simulink model "sldrt_newtest_2025b"  (R2025b)
settings: Solver=FixedStepDiscrete  StartTime=0.0  StopTime=inf  FixedStep=0.02  RelTol=1e-3  EnableMultiTasking=on
PreLoadFcn:
  | setup_buses
  | FromApp_Template = Simulink.Bus.createMATLABStruct('FromAppBus_Type');
  | assignin('base', 'FromApp_Template', FromApp_Template);
model workspace (MAT data in the model file):
  AppAirBtn = Simulink.Parameter
  AppAirBtn.Value = 0
  AppAirBtn.Complexity = 'real'
  AppAirBtn.Dimensions = [1 1]
  AppAirBtn.DataType = 'boolean'
  AppAmplitude = Simulink.Parameter
  AppAmplitude.Value = 800
  AppAmplitude.Complexity = 'real'
  AppAmplitude.Dimensions = [1 1]
  AppAmplitude.DataType = 'auto'
  AppPeriods = Simulink.Parameter
  AppPeriods.Value = 2
  AppPeriods.Complexity = 'real'
  AppPeriods.Dimensions = [1 1]
  AppPeriods.DataType = 'auto'
  AppSharpness = Simulink.Parameter
  AppSharpness.Value = 2
  AppSharpness.Complexity = 'real'
  AppSharpness.Dimensions = [1 1]
  AppSharpness.DataType = 'auto'
  AppZeroBtn = Simulink.Parameter
  AppZeroBtn.Value = 0
  AppZeroBtn.Complexity = 'real'
  AppZeroBtn.Dimensions = [1 1]
  AppZeroBtn.DataType = 'boolean'
  Code = Simulink.Parameter
  Code.Value = 279.564441178
  Code.Complexity = 'real'
  Code.Dimensions = [1 1]
  Code.DataType = 'auto'
  CodeScaleCoeff = Simulink.Parameter
  CodeScaleCoeff.Value = 0.0214546484044
  CodeScaleCoeff.Complexity = 'real'
  CodeScaleCoeff.Dimensions = [1 1]
  CodeScaleCoeff.DataType = 'auto'
  SignalToDAC = Simulink.Parameter
  SignalToDAC.Value = [2048 2048 2049 2049 2050 2050 2050 2051 2051 2051 2052 2052 ... (20000 elements, 1x20000)]
  SignalToDAC.Complexity = 'real'
  SignalToDAC.Dimensions = [1 20000]
  SignalToDAC.DataType = 'uint16'
  myLUTobj = Simulink.LookupTable
  myLUTobj.Table = Simulink.lookuptable.Table
  myLUTobj.Table.Value = [1 2 3 4 5 6 7 8 9 10]
  myLUTobj.Table.Dimensions = [1 10]
  myLUTobj.Table.DataType = 'auto'
  myLUTobj.Table.FieldName = 'V'
  myLUTobj.Breakpoints = Simulink.lookuptable.Breakpoint
  myLUTobj.Breakpoints.Value = [1 2 3 4 5 6 7 8 9 10]
  myLUTobj.Breakpoints.TunableSizeName = 'N1'
  myLUTobj.Breakpoints.TunableSizeValue = -1
  myLUTobj.Breakpoints.Dimensions = [1 10]
  myLUTobj.Breakpoints.DataType = 'auto'
  myLUTobj.Breakpoints.FieldName = 'Value'
  myLUTobj.AllowMultipleInstancesOfTypeToHaveDifferentTableBreakpointSizes = 0
  myLUTobj.SupportTunableSize = 1
  myLUTobj.StructTypeInfo = Simulink.lookuptable.StructTypeInfo
  myLUTobj.StructTypeInfo.Name = 'myLUTstruct'
  myLUTobj.StructTypeInfo.DataScope = 'Auto'
  xx = Simulink.Parameter
  xx.Value = [41343 41343.1 41343.2 41343.3 41343.4 41343.5 41343.6 41343.7 41343.8 41343.9 41344 41682 41973 42429 43533 44717 46388 47769 49334 50678 51343 53185 55663 57862 60000]
  xx.Complexity = 'real'
  xx.Dimensions = [1 25]
  xx.DataType = 'auto'
  yy = Simulink.Parameter
  yy.Value = [3122 3121.9 3121.8 3121.7 3121.6 3121.5 3121.4 3121.3 3121.2 3121.1 3121 2440 1964 1465 976 698 466 335 232 181 154 103 51 20 0]
  yy.Complexity = 'real'
  yy.Dimensions = [1 25]
  yy.DataType = 'auto'
libraries: simulink x7, simulink_extras x4, dspnetwork x2, dspstat3 x2, etargetslib x1
settings Model: ExplicitPartitioning=on  Creator=Huawei  LastModifiedBy=lolve
settings SolverCC: AlgebraicLoopSolver=TrustRegion  AutoInsertRateTranBlk=on  DecoupledContinuousIntegration=on  MinimalZcImpactIntegration=on
settings DataIOCC: ExternalInput=TestInput
settings OptimizationCC: BlockReduction=off  DefaultParameterBehavior=Inlined  UseDivisionForNetSlopeComputation=on  GainParamInheritBuiltInType=on  UseFloatMulNetSlope=on  InlineInvariantSignals=on  OptimizeBlockIOStorage=off  BufferReuse=off  ReuseModelBlockBuffer=off  GlobalBufferReuse=off  ExpressionFolding=off  EnableMemcpy=off  PassReuseOutputArgsThreshold=0.0  LocalBlockOutputs=off  EfficientFloat2IntCast=on  MaxStackSize=64  OptimizeDataStoreBuffers=off  BusAssignmentInplaceUpdate=off  OptimizationLevel=level0  OptimizationCustomize=off
settings DebuggingCC: ParameterTunabilityLossMsg=error  UnconnectedInputMsg=warning  UnconnectedOutputMsg=warning  UnconnectedLineMsg=warning  ArithmeticOperatorsInVariantConditions=warning
settings HardwareCC: ProdBitPerLong=64.0  ProdHWDeviceType=Intel->x86-64 (Linux 64)
settings ModelReferenceCC: EnableRefExpFcnMdlSchedulingChecks=on
settings SFSimCC: SimUseLocalCustomCode=off  MATLABDynamicMemAlloc=off  CustomCodeUndefinedFunction=UseInterfaceOnly
settings RTWCC: SystemTargetFile=sldrt.tlc  TemplateMakefile=sldrt.tmf  GenerateReport=on  RTWUseLocalCustomCode=off  Toolchain=Microsoft Visual C++ 2022 v17.0 | nmake (64-bit Windows)  LaunchReport=on  RTWCompilerOptimization=on  GPUComputeCapability=3.5  DLArmComputeVersion=19.05  Description=Simulink Desktop Real-Time
settings CodeAppCC: ForceParamTrailComments=on  MaxIdLength=95.0  OperatorAnnotations=on
settings SimulinkDesktopRealTimeCC: ExtModeTransport=0.0  ExtModeStaticAllocSize=1000000.0  TargetLibSuffix=_sldrt.a  TargetPreCompLibLocation=D:\MATLAB\R2025b\toolbox\sldrt\lib\win64  MultiwordLength=2048.0  DynamicStringBufferSize=256.0  ParMdlRefBuildCompliant=on  PreserveMATLABNamespacesInGeneratedCode=on  SubcomponentCodeInterfacePackaging=Reusable function

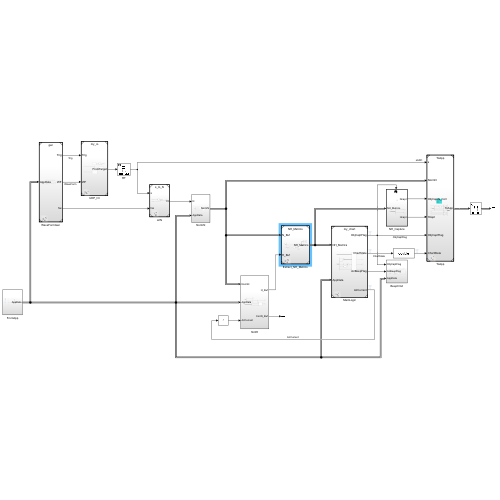
[thumbnail: Simulink's stored preview of the top-level diagram]
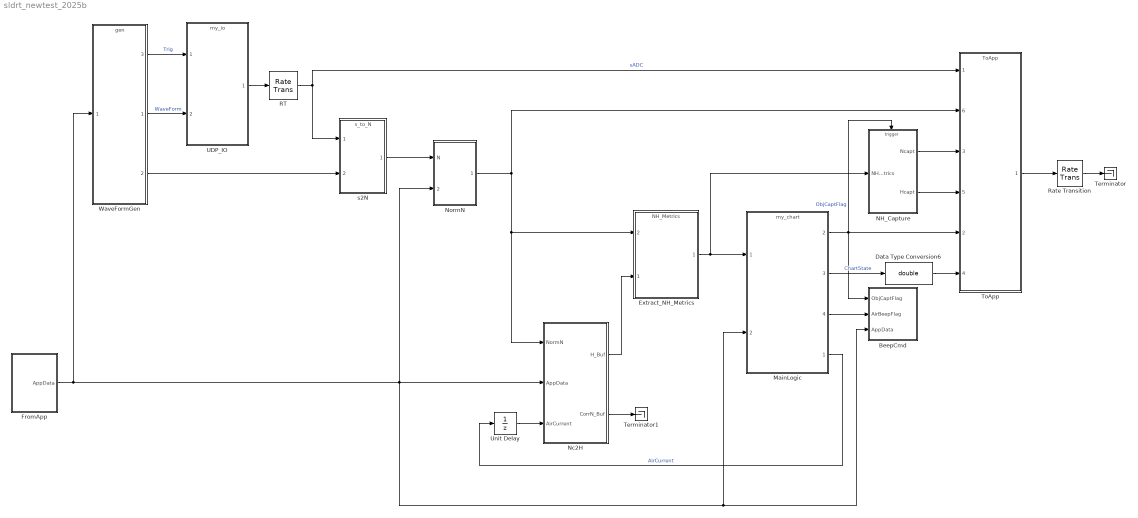
== system sldrt_newtest_2025b ==
  BeepCmd : Subsystem
  Data Type Conversion6 : DataTypeConversion  OutDataTypeStr=double  SaturateOnIntegerOverflow=off  RndMeth=Floor
  Extract_NH_Metrics : ModelReference  ModelNameDialog=NH_Metrics  SimulationMode=Normal  ModelReferenceVersion=1.50
      settings: PortSchema="{\"entries\":[{\"content\":{\"sides\":[{\"content\":{\"connectorIds\":[\"In2\",\"In1\"]},\"type\":\"ConnectorPlacement.EquallySpacedRectSide\",\"uuid\":\"3a38ccda-2223-4b10-94c8-e18dfc340c6f\"},{\"content\":{\"connectorIds\":[\"Out1\"],\"side\":\"RIGHT\"},\"type\":\"ConnectorPlacement.EquallySpacedRectSide\",\"uuid\":\"8419e0ff-c5db-4e1e-bcd8-780560147c58\"},{\"content\":{\"side\":\"TOP\"},\"type\":\"ConnectorPlacement.EquallySpacedRectSide\",\"uuid\":\"08e19ae9-9d85-4fd9-806d-4003401e858c\"}]},\"type\":\"ConnectorPlacement.EquallySpacedConnector\",\"uuid\":\"799394af-d852-43f2-8721-bc316fb3f3ae\"}],\"packageUris\":[\"http://schema.mathworks.com/mf0/Connector/R2020b\"],\"version\":\"1.0\"}"
  FromApp : Subsystem
  MainLogic : ModelReference  Priority=2  ModelNameDialog=my_chart.slx  SimulationMode=Normal  ScheduleRatesWith=Schedule Editor  ModelReferenceVersion=1.246
      settings: PortSchema="{\"entries\":[{\"content\":{\"sides\":[{\"content\":{\"connectorIds\":[\"In1\",\"In2\"]},\"type\":\"ConnectorPlacement.EquallySpacedRectSide\",\"uuid\":\"0ee1a6e0-4898-4e5e-a3f2-a4873c516c9b\"},{\"content\":{\"connectorIds\":[\"Out2\",\"Out3\",\"Out4\",\"Out1\"],\"side\":\"RIGHT\"},\"type\":\"ConnectorPlacement.EquallySpacedRectSide\",\"uuid\":\"631dc309-49f9-48aa-93e0-96384f954726\"},{\"content\":{\"side\":\"TOP\"},\"type\":\"ConnectorPlacement.EquallySpacedRectSide\",\"uuid\":\"941348e0-d81f-4f79-b9d4-bd78ea26c6c3\"}]},\"type\":\"ConnectorPlacement.EquallySpacedConnector\",\"uuid\":\"94e2f426-079c-4c5f-a540-67617520c55b\"}],\"packageUris\":[\"http://schema.mathworks.com/mf0/Connector/R2020b\"],\"version\":\"1.0\"}"
  NH_Capture : Subsystem
  Nc2H : Subsystem
  NormN : Subsystem
  RT : RateTransition  Integrity=off  Deterministic=off  OutPortSampleTime=0.02
  Rate Transition : RateTransition
  Terminator : Terminator
  Terminator1 : Terminator
  ToApp : ModelReference  ModelNameDialog=ToApp.slx  SimulationMode=Normal  ModelReferenceVersion=1.41
      settings: PortSchema="{\"entries\":[{\"content\":{\"sides\":[{\"content\":{\"connectorIds\":[\"In1\",\"In6\",\"In3\",\"In5\",\"In2\",\"In4\"]},\"type\":\"ConnectorPlacement.EquallySpacedRectSide\",\"uuid\":\"2a60f3ad-f22a-481e-bfa0-3f1feb70fa0e\"},{\"content\":{\"connectorIds\":[\"Out1\"],\"side\":\"RIGHT\"},\"type\":\"ConnectorPlacement.EquallySpacedRectSide\",\"uuid\":\"a97ccfa7-4022-4d86-888c-0861d8007155\"},{\"content\":{\"side\":\"TOP\"},\"type\":\"ConnectorPlacement.EquallySpacedRectSide\",\"uuid\":\"d2721f0e-98b2-48c2-b67a-f5bd578bfe97\"}]},\"type\":\"ConnectorPlacement.EquallySpacedConnector\",\"uuid\":\"dadb772c-2c9f-4732-9bcd-da2802ebc2cf\"}],\"packageUris\":[\"http://schema.mathworks.com/mf0/Connector/R2020b\"],\"version\":\"1.0\"}"
  UDP_IO : ModelReference  ModelNameDialog=my_io.slx  SimulationMode=Normal  ModelReferenceVersion=1.32
  Unit Delay : UnitDelay  InitialCondition=1  SampleTime=-1  HasFrameUpgradeWarning=on
  WaveFormGen : ModelReference  ModelNameDialog=gen.slx  SimulationMode=Normal  ModelReferenceVersion=1.31
      settings: PortSchema="{\"entries\":[{\"content\":{\"sides\":[{\"content\":{\"connectorIds\":[\"In1\"]},\"type\":\"ConnectorPlacement.EquallySpacedRectSide\",\"uuid\":\"6ec36bc1-2d75-43bf-b54c-2c7b61273d73\"},{\"content\":{\"connectorIds\":[\"Out3\",\"Out1\",\"Out2\"],\"side\":\"RIGHT\"},\"type\":\"ConnectorPlacement.EquallySpacedRectSide\",\"uuid\":\"17382908-6507-41c0-8990-8a468161a0d7\"},{\"content\":{\"side\":\"TOP\"},\"type\":\"ConnectorPlacement.EquallySpacedRectSide\",\"uuid\":\"0c9326df-e88c-4f4a-83e1-d6c039129936\"}]},\"type\":\"ConnectorPlacement.EquallySpacedConnector\",\"uuid\":\"e56dde6f-bf8e-407c-8fff-cfa8939317ce\"}],\"packageUris\":[\"http://schema.mathworks.com/mf0/Connector/R2020b\"],\"version\":\"1.0\"}"
  s2N : ModelReference  ModelNameDialog=s_to_N.slx  SimulationMode=Normal  ModelReferenceVersion=1.5
  wires:
  UDP_IO/1 -> RT/1
  WaveFormGen/1 -> UDP_IO/2  "WaveForm"
  WaveFormGen/2 -> s2N/2
  MainLogic/1 -> Unit Delay/1  "AirCurrent"
  RT/1 -> s2N/1, ToApp/1  "sADC"
  ToApp/1 -> Rate Transition/1
  Rate Transition/1 -> Terminator/1
  s2N/1 -> NormN/1(N)
  Unit Delay/1 -> Nc2H/3(AirCurrent)
  MainLogic/2 -> BeepCmd/1(ObjCaptFlag), NH_Capture/Trigger, ToApp/2  "ObjCaptFlag"
  NH_Capture/1(Ncapt) -> ToApp/3
  MainLogic/3 -> Data Type Conversion6/1  "ChartState"
  Extract_NH_Metrics/1 -> NH_Capture/1(NH_Metrics), MainLogic/1
  NH_Capture/2(Hcapt) -> ToApp/5
  Nc2H/2(CorrN_Buf) -> Terminator1/1
  WaveFormGen/3 -> UDP_IO/1  "Trig"
  FromApp/1(AppData) -> WaveFormGen/1, MainLogic/2, BeepCmd/3(AppData), NormN/2(AppData), Nc2H/2(AppData)
  MainLogic/4 -> BeepCmd/2(AirBeepFlag)
  NormN/1(NormN) -> Nc2H/1(NormN), Extract_NH_Metrics/2, ToApp/6
  Nc2H/1(H_Buf) -> Extract_NH_Metrics/1
  Data Type Conversion6/1 -> ToApp/4

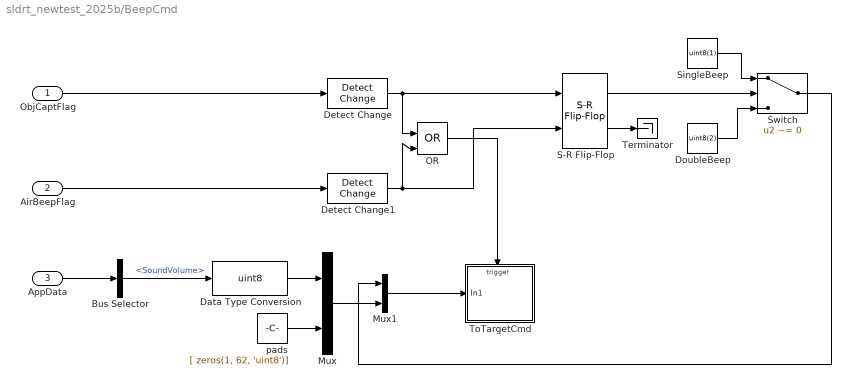
== system sldrt_newtest_2025b/BeepCmd ==
  ObjCaptFlag : Inport  OutDataTypeStr=boolean  PortDimensions=1
  AirBeepFlag : Inport  Port=2  OutDataTypeStr=boolean  PortDimensions=1
  AppData : Inport  Port=3  OutDataTypeStr=Bus: FromAppBus_Type  PortDimensions=1
  Bus Selector : BusSelector  OutputSignals=SoundVolume
  Data Type Conversion : DataTypeConversion  OutDataTypeStr=uint8  SaturateOnIntegerOverflow=off  RndMeth=Floor
  Detect Change : simulink/Logic and Bit Operations/Detect Change  vinit=0  OutDataTypeStr=boolean
  Detect Change1 : simulink/Logic and Bit Operations/Detect Change  vinit=0  OutDataTypeStr=boolean
  DoubleBeep : Constant  Value=uint8(2)  OutDataTypeStr=uint8
  Mux : Mux  Inputs=2
  Mux1 : Mux  Inputs=2
  OR : Logic  Operator=OR  IconShape=distinctive  AllPortsSameDT=off  OutDataTypeStr=boolean
  S-R Flip-Flop : simulink_extras/Flip Flops/S-R Flip-Flop  initial_condition=0
  SingleBeep : Constant  Value=uint8(1)  OutDataTypeStr=uint8
  Switch : Switch  Criteria=u2 ~= 0  SaturateOnIntegerOverflow=off  InputSameDT=off
  Terminator : Terminator
  ToTargetCmd : Subsystem
  pads : Constant  Value=[ zeros(1, 62, 'uint8')]  OutDataTypeStr=uint8
  wires:
  S-R Flip-Flop/1 -> Switch/2
  Switch/1 -> Mux1/1
  DoubleBeep/1 -> Switch/3
  ObjCaptFlag/1 -> Detect Change/1
  Detect Change1/1 -> OR/2, S-R Flip-Flop/2
  S-R Flip-Flop/2 -> Terminator/1
  SingleBeep/1 -> Switch/1
  OR/1 -> ToTargetCmd/Trigger
  Detect Change/1 -> S-R Flip-Flop/1, OR/1
  AirBeepFlag/1 -> Detect Change1/1
  AppData/1 -> Bus Selector/1
  Bus Selector/1 -> Data Type Conversion/1  "<SoundVolume>"
  Data Type Conversion/1 -> Mux/1
  pads/1 -> Mux/2
  Mux/1 -> Mux1/2
  Mux1/1 -> ToTargetCmd/1(In1)

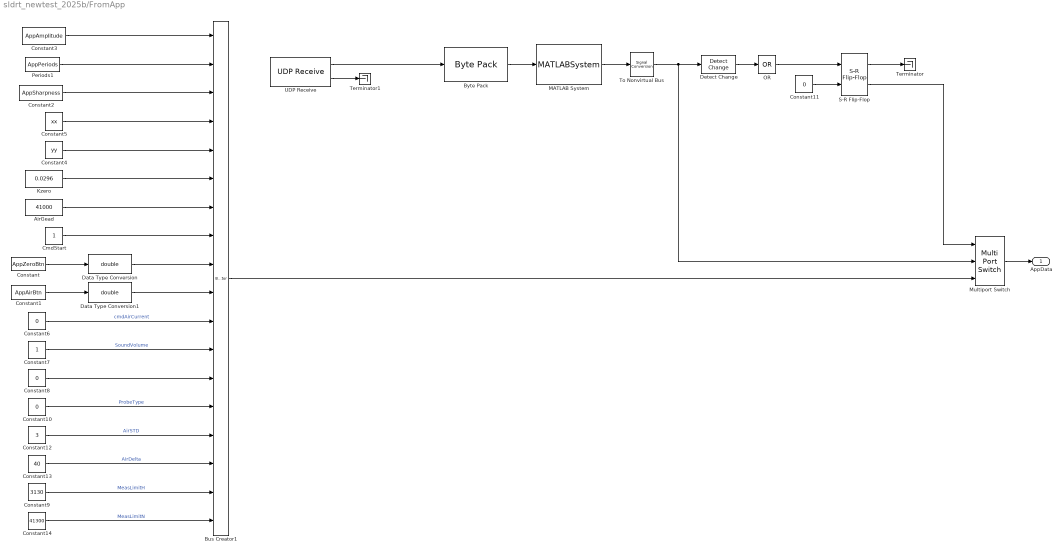
== system sldrt_newtest_2025b/FromApp ==
  AirGead : Constant  Value=41000  OutDataTypeStr=double
  Bus Creator1 : BusCreator  Inputs=18  OutDataTypeStr=Bus: FromAppBus_Type
      settings: InheritFromInputs=off
  Byte Pack : etargetslib/Byte Pack  datatypes={'double'}  byteAlign=1
  CmdStart : Constant  OutDataTypeStr=double
  Constant : Constant  Value=AppZeroBtn  OutDataTypeStr=boolean
  Constant1 : Constant  Value=AppAirBtn  OutDataTypeStr=boolean
  Constant10 : Constant  Value=0
  Constant11 : Constant  Value=0  OutDataTypeStr=boolean
  Constant12 : Constant  Value=3
  Constant13 : Constant  Value=40
  Constant14 : Constant  Value=41300
  Constant2 : Constant  Value=AppSharpness
  Constant3 : Constant  Value=AppAmplitude
  Constant4 : Constant  Value=yy
  Constant5 : Constant  Value=xx
  Constant6 : Constant  Value=0
  Constant7 : Constant
  Constant8 : Constant  Value=0
  Constant9 : Constant  Value=3130
  Data Type Conversion : DataTypeConversion  OutDataTypeStr=double  SaturateOnIntegerOverflow=off  RndMeth=Floor
  Data Type Conversion1 : DataTypeConversion  OutDataTypeStr=double  SaturateOnIntegerOverflow=off  RndMeth=Floor
  Detect Change : simulink/Logic and Bit Operations/Detect Change  vinit=0  OutDataTypeStr=boolean
  Kzero : Constant  Value=0.0296  OutDataTypeStr=double
  MATLAB System : MATLABSystem  System=FromAppParser  TemplateStructure=FromApp_Template  SimulateUsing=Interpreted execution
      mask Type: FromAppParser
  Multiport Switch : MultiPortSwitch  DataPortOrder=Zero-based contiguous  Inputs=2  zeroidx=on  SaturateOnIntegerOverflow=off  InputSameDT=off
  OR : Logic  Operator=OR  Inputs=1  IconShape=distinctive  AllPortsSameDT=off  OutDataTypeStr=boolean
  Periods1 : Constant  Value=AppPeriods
  S-R Flip-Flop : simulink_extras/Flip Flops/S-R Flip-Flop  initial_condition=0
  Terminator : Terminator
  Terminator1 : Terminator
  To Nonvirtual Bus : SignalConversion  ConversionOutput=Virtual bus  OverrideOpt=off
  UDP Receive : dspnetwork/UDP Receive  localURL='0.0.0.0'  localPort=25010  remoteURL='0.0.0.0'  remotePort=-1  recvBufferSize=2048  dims=128  signalDatatype=double  isComplex=off  isVarSize=off  showBlockingTime=off  blockingTime=0  sampletime=0.02  blockPlatform=[]
      settings: LibrarySourceBlock=dspsrcs4/UDP Receive
  AppData : Outport  OutDataTypeStr=Bus: FromAppBus_Type  PortDimensions=1
  wires:
  UDP Receive/2 -> Terminator1/1
  MATLAB System/1 -> To Nonvirtual Bus/1
  Constant/1 -> Data Type Conversion/1
  Constant1/1 -> Data Type Conversion1/1
  Constant3/1 -> Bus Creator1/1
  Periods1/1 -> Bus Creator1/2
  Constant2/1 -> Bus Creator1/3
  Constant5/1 -> Bus Creator1/4
  Constant4/1 -> Bus Creator1/5
  Kzero/1 -> Bus Creator1/6
  AirGead/1 -> Bus Creator1/7
  CmdStart/1 -> Bus Creator1/8
  Data Type Conversion/1 -> Bus Creator1/9
  Data Type Conversion1/1 -> Bus Creator1/10
  Constant6/1 -> Bus Creator1/11  "cmdAirCurrent"
  Constant7/1 -> Bus Creator1/12  "SoundVolume"
  Constant8/1 -> Bus Creator1/13
  Bus Creator1/1 -> Multiport Switch/3
  Multiport Switch/1 -> AppData/1
  S-R Flip-Flop/2 -> Multiport Switch/1
  Detect Change/1 -> OR/1
  Constant11/1 -> S-R Flip-Flop/2
  OR/1 -> S-R Flip-Flop/1
  S-R Flip-Flop/1 -> Terminator/1
  Constant10/1 -> Bus Creator1/14  "ProbeType"
  To Nonvirtual Bus/1 -> Multiport Switch/2, Detect Change/1
  Constant12/1 -> Bus Creator1/15  "AirSTD"
  Constant13/1 -> Bus Creator1/16  "AirDelta"
  UDP Receive/1 -> Byte Pack/1
  Byte Pack/1 -> MATLAB System/1
  Constant9/1 -> Bus Creator1/17  "MeasLimitH"
  Constant14/1 -> Bus Creator1/18  "MeasLimitN"

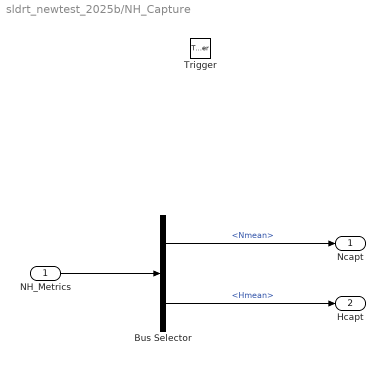
== system sldrt_newtest_2025b/NH_Capture ==
  NH_Metrics : Inport  OutDataTypeStr=Bus: NH_MetricsBus_Type
  Trigger : TriggerPort  TriggerType=either  VariantControl=(inherit)  PortDimensions=1
  Bus Selector : BusSelector  OutputSignals=Nmean,Hmean
  Ncapt : Outport  OutDataTypeStr=double  PortDimensions=1
  Hcapt : Outport  Port=2  OutDataTypeStr=double  PortDimensions=1
  wires:
  NH_Metrics/1 -> Bus Selector/1
  Bus Selector/2 -> Hcapt/1  "<Hmean>"
  Bus Selector/1 -> Ncapt/1  "<Nmean>"

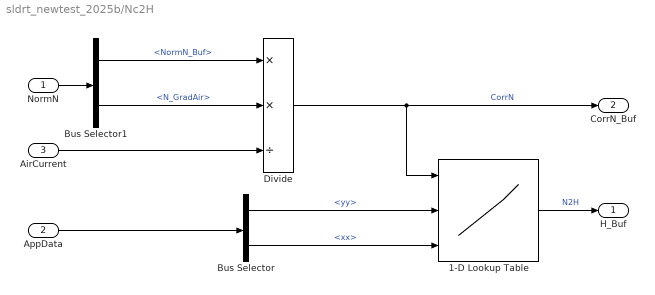
== system sldrt_newtest_2025b/Nc2H ==
  NormN : Inport  OutDataTypeStr=Bus: N_Bus_Type  PortDimensions=1
  AppData : Inport  Port=2  OutDataTypeStr=Bus: FromAppBus_Type  PortDimensions=1
  AirCurrent : Inport  Port=3
  1-D Lookup Table : Lookup_n-D  NumberOfTableDimensions=1  LookupTableObject=myLUTobj  BreakpointsForDimension1Source=Input port  BreakpointsForDimension1=xx  IndexSearchMethod=Linear search  TableSource=Input port  Table=yy  InternalRulePriority=Speed  RndMeth=Simplest
      settings: InputPortMap=u0,p221,p5
  Bus Selector : BusSelector  OutputSignals=yy,xx
  Bus Selector1 : BusSelector  OutputSignals=NormN_Buf,N_GradAir
  Divide : Product  Inputs=**/
  H_Buf : Outport
  CorrN_Buf : Outport  Port=2  OutDataTypeStr=double
  wires:
  Divide/1 -> CorrN_Buf/1, 1-D Lookup Table/1  "CorrN"
  AirCurrent/1 -> Divide/3
  Bus Selector/1 -> 1-D Lookup Table/2  "<yy>"
  Bus Selector1/1 -> Divide/1  "<NormN_Buf>"
  1-D Lookup Table/1 -> H_Buf/1  "N2H"
  Bus Selector/2 -> 1-D Lookup Table/3  "<xx>"
  Bus Selector1/2 -> Divide/2  "<N_GradAir>"
  AppData/1 -> Bus Selector/1
  NormN/1 -> Bus Selector1/1

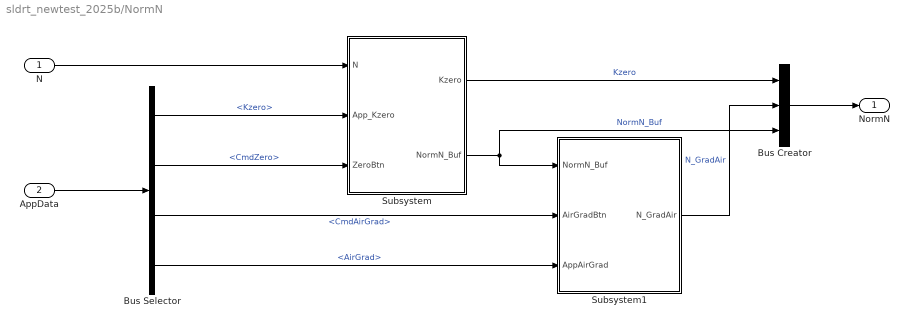
== system sldrt_newtest_2025b/NormN ==
  N : Inport
  AppData : Inport  Port=2  OutDataTypeStr=Bus: FromAppBus_Type  PortDimensions=1
  Bus Creator : BusCreator  Inputs=3  OutDataTypeStr=Bus: N_Bus_Type
      settings: InheritFromInputs=off
  Bus Selector : BusSelector  OutputSignals=Kzero,CmdZero,CmdAirGrad,AirGrad
  Subsystem : Subsystem
  Subsystem1 : Subsystem
  NormN : Outport  OutDataTypeStr=Bus: N_Bus_Type
  wires:
  Bus Selector/2 -> Subsystem/3(ZeroBtn)  "<CmdZero>"
  Subsystem/2(NormN_Buf) -> Bus Creator/3, Subsystem1/1(NormN_Buf)  "NormN_Buf"
  Bus Selector/3 -> Subsystem1/2(AirGradBtn)  "<CmdAirGrad>"
  Subsystem1/1(N_GradAir) -> Bus Creator/2  "N_GradAir"
  N/1 -> Subsystem/1(N)
  Subsystem/1(Kzero) -> Bus Creator/1  "Kzero"
  Bus Selector/4 -> Subsystem1/3(AppAirGrad)  "<AirGrad>"
  Bus Selector/1 -> Subsystem/2(App_Kzero)  "<Kzero>"
  AppData/1 -> Bus Selector/1
  Bus Creator/1 -> NormN/1

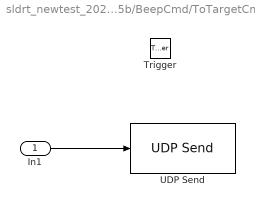
== system sldrt_newtest_2025b/BeepCmd/ToTargetCmd ==
  In1 : Inport
  Trigger : TriggerPort  VariantControl=(inherit)  PortDimensions=1
  UDP Send : dspnetwork/UDP Send  remoteURL='127.0.0.1'  remotePort=25003  localURL='0.0.0.0'  localPortSource=Specify via dialog  localPort=25006  sendBufferSize=64  sampletime=-1  blockPlatform=[]  separateLengthPort=0
      settings: LibrarySourceBlock=dspsnks4/UDP Send
  wires:
  In1/1 -> UDP Send/1

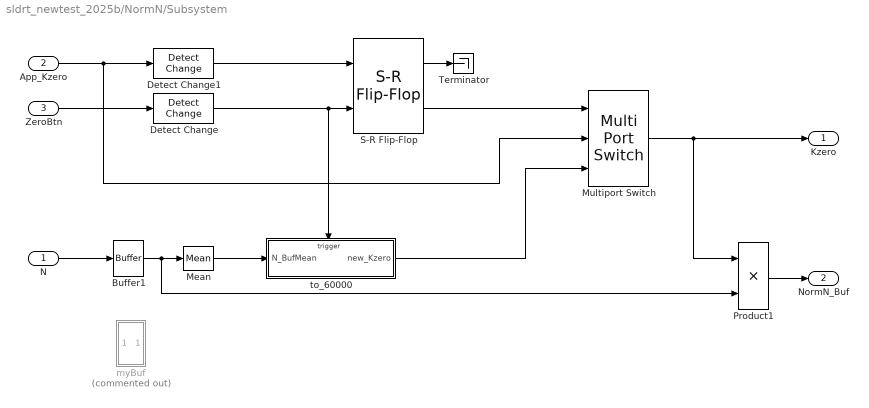
== system sldrt_newtest_2025b/NormN/Subsystem ==
  N : Inport
  App_Kzero : Inport  Port=2  OutDataTypeStr=double  PortDimensions=1
  ZeroBtn : Inport  Port=3
  Buffer1 : Buffer  N=16  V=15  OutputFrames=off
  Detect Change : simulink/Logic and Bit Operations/Detect Change  vinit=0  OutDataTypeStr=boolean
  Detect Change1 : simulink/Logic and Bit Operations/Detect Change  vinit=0  OutDataTypeStr=boolean
  Mean : dspstat3/Mean  run=off  InputProcessing=Columns as channels (frame based)  reset_popup=None  directionMode=Each column  dimension=1  roiEnable=off  roiType=Rectangles  roiPortion=Entire ROI  roiOutput=Individual statistics for each ROI  roiFlag=off  roundingMode=Floor  overflowMode=off  outputDataTypeStr=Inherit: Same as accumulator  outputMin=[]  outputMax=[]  outputLastDataTypeStr=Inherit: Same as accumulator
  Multiport Switch : MultiPortSwitch  DataPortOrder=Zero-based contiguous  Inputs=2  zeroidx=on  OutDataTypeStr=double  SaturateOnIntegerOverflow=off  InputSameDT=off
  Product1 : Product
  S-R Flip-Flop : simulink_extras/Flip Flops/S-R Flip-Flop  initial_condition=0
  Terminator : Terminator
  myBuf : Subsystem  Commented=on
  to_60000 : Subsystem
  Kzero : Outport  OutDataTypeStr=double  PortDimensions=1
  NormN_Buf : Outport  Port=2
  wires:
  Product1/1 -> NormN_Buf/1
  Buffer1/1 -> Product1/2, Mean/1
  Mean/1 -> to_60000/1(N_BufMean)
  N/1 -> Buffer1/1
  to_60000/1(new_Kzero) -> Multiport Switch/3
  ZeroBtn/1 -> Detect Change/1
  Detect Change/1 -> S-R Flip-Flop/2, to_60000/Trigger
  App_Kzero/1 -> Multiport Switch/2, Detect Change1/1
  Detect Change1/1 -> S-R Flip-Flop/1
  S-R Flip-Flop/2 -> Multiport Switch/1
  S-R Flip-Flop/1 -> Terminator/1
  Multiport Switch/1 -> Product1/1, Kzero/1

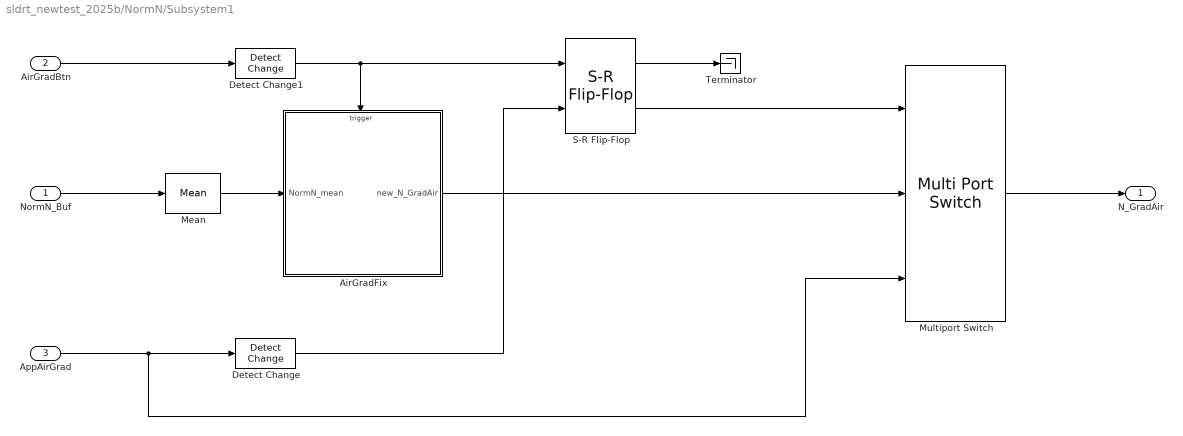
== system sldrt_newtest_2025b/NormN/Subsystem1 ==
  NormN_Buf : Inport
  AirGradBtn : Inport  Port=2
  AppAirGrad : Inport  Port=3
  AirGradFix : Subsystem  TreatAsAtomicUnit=on
  Detect Change : simulink/Logic and Bit Operations/Detect Change  vinit=0  OutDataTypeStr=boolean
      settings: LibrarySourceBlock=|
      | hdlsllib/Logic and Bit
      | Operations/Detect
      | Change
  Detect Change1 : simulink/Logic and Bit Operations/Detect Change  vinit=0  OutDataTypeStr=boolean
      settings: LibrarySourceBlock=|
      | hdlsllib/Logic and Bit
      | Operations/Detect
      | Change
  Mean : dspstat3/Mean  run=off  InputProcessing=Columns as channels (frame based)  reset_popup=None  directionMode=Each column  dimension=1  roiEnable=off  roiType=Rectangles  roiPortion=Entire ROI  roiOutput=Individual statistics for each ROI  roiFlag=off  roundingMode=Floor  overflowMode=off  outputDataTypeStr=Inherit: Same as accumulator  outputMin=[]  outputMax=[]  outputLastDataTypeStr=Inherit: Same as accumulator
  Multiport Switch : MultiPortSwitch  DataPortOrder=Zero-based contiguous  Inputs=2  zeroidx=on  OutDataTypeStr=double  SaturateOnIntegerOverflow=off  InputSameDT=off
  S-R Flip-Flop : simulink_extras/Flip Flops/S-R Flip-Flop  initial_condition=0
  Terminator : Terminator
  N_GradAir : Outport  OutDataTypeStr=double
  wires:
  AirGradBtn/1 -> Detect Change1/1
  NormN_Buf/1 -> Mean/1
  AppAirGrad/1 -> Multiport Switch/3, Detect Change/1
  Multiport Switch/1 -> N_GradAir/1
  Mean/1 -> AirGradFix/1(NormN_mean)
  Detect Change1/1 -> AirGradFix/Trigger, S-R Flip-Flop/1
  Detect Change/1 -> S-R Flip-Flop/2
  S-R Flip-Flop/1 -> Terminator/1
  AirGradFix/1(new_N_GradAir) -> Multiport Switch/2
  S-R Flip-Flop/2 -> Multiport Switch/1

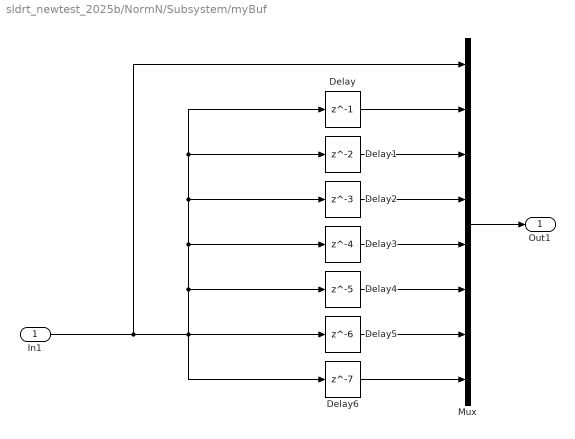
== system sldrt_newtest_2025b/NormN/Subsystem/myBuf ==
  In1 : Inport
  Delay : Delay  DelayLength=1  InputProcessing=Columns as channels (frame based)
  Delay1 : Delay  InputProcessing=Columns as channels (frame based)
  Delay2 : Delay  DelayLength=3  InputProcessing=Columns as channels (frame based)
  Delay3 : Delay  DelayLength=4  InputProcessing=Columns as channels (frame based)
  Delay4 : Delay  DelayLength=5  InputProcessing=Columns as channels (frame based)
  Delay5 : Delay  DelayLength=6  InputProcessing=Columns as channels (frame based)
  Delay6 : Delay  DelayLength=7  InputProcessing=Columns as channels (frame based)
  Mux : Mux  Inputs=8
  Out1 : Outport
  wires:
  In1/1 -> Mux/1, Delay6/1, Delay4/1, Delay3/1, Delay2/1, Delay1/1, Delay/1, Delay5/1
  Delay/1 -> Mux/2
  Delay1/1 -> Mux/3
  Delay2/1 -> Mux/4
  Delay3/1 -> Mux/5
  Delay4/1 -> Mux/6
  Delay5/1 -> Mux/7
  Delay6/1 -> Mux/8
  Mux/1 -> Out1/1

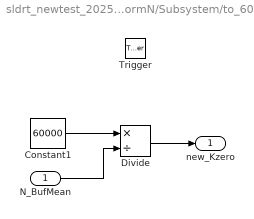
== system sldrt_newtest_2025b/NormN/Subsystem/to_60000 ==
  N_BufMean : Inport
  Trigger : TriggerPort  VariantControl=(inherit)  InitialTriggerSignalState=zero  PortDimensions=1
  Constant1 : Constant  Value=60000  SampleTime=-1
  Divide : Product  Inputs=*/
  new_Kzero : Outport  InitialOutput=1
  wires:
  Constant1/1 -> Divide/1
  N_BufMean/1 -> Divide/2
  Divide/1 -> new_Kzero/1

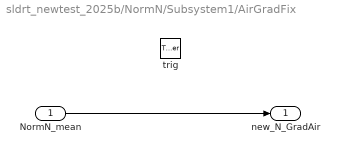
== system sldrt_newtest_2025b/NormN/Subsystem1/AirGradFix ==
  NormN_mean : Inport  OutDataTypeStr=double  PortDimensions=1
  trig : TriggerPort  VariantControl=(inherit)  InitialTriggerSignalState=zero
  new_N_GradAir : Outport  OutDataTypeStr=double  PortDimensions=1  InitialOutput=0
  wires:
  NormN_mean/1 -> new_N_GradAir/1
